simulink model "TST_Tra_Add"  (R2016b)
settings: Solver=FixedStepDiscrete  StartTime=0.0  StopTime=simTime  FixedStep=sampleTime  RelTol=1e-3
values from neighbouring files (symbols this model uses):
  testCase = 1    [initTST_Tra_Add_001.m]    (also in initTST_Tra_Add_002.m = 2)
libraries: simulink x7, UnitTest_Lib x4
settings Model: Creator=zhengjinyan  LastModifiedBy=zhengjinyan
settings DebuggingCC: SignalRangeChecking=error

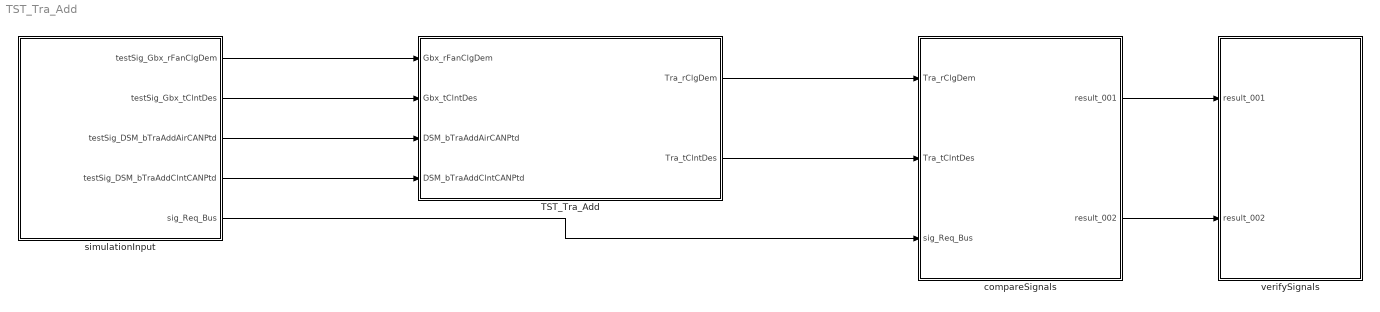
== system TST_Tra_Add ==
  TST_Tra_Add : Subsystem
  compareSignals : Subsystem
  simulationInput : Subsystem
  verifySignals : Subsystem
  wires:
  simulationInput/1(testSig_Gbx_rFanClgDem) -> TST_Tra_Add/1(Gbx_rFanClgDem)
  simulationInput/2(testSig_Gbx_tClntDes) -> TST_Tra_Add/2(Gbx_tClntDes)
  simulationInput/3(testSig_DSM_bTraAddAirCANPtd) -> TST_Tra_Add/3(DSM_bTraAddAirCANPtd)
  simulationInput/4(testSig_DSM_bTraAddClntCANPtd) -> TST_Tra_Add/4(DSM_bTraAddClntCANPtd)
  TST_Tra_Add/1(Tra_rClgDem) -> compareSignals/1(Tra_rClgDem)
  TST_Tra_Add/2(Tra_tClntDes) -> compareSignals/2(Tra_tClntDes)
  simulationInput/5(sig_Req_Bus) -> compareSignals/3(sig_Req_Bus)
  compareSignals/1(result_001) -> verifySignals/1(result_001)
  compareSignals/2(result_002) -> verifySignals/2(result_002)

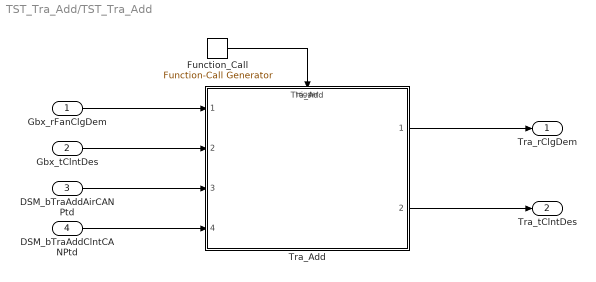
== system TST_Tra_Add/TST_Tra_Add ==
  Gbx_rFanClgDem : Inport
  Gbx_tClntDes : Inport  Port=2
  DSM_bTraAddAirCANPtd : Inport  Port=3
  DSM_bTraAddClntCANPtd : Inport  Port=4
  Function_Call : simulink/Ports & Subsystems/Function-Call Generator  sample_time=sampleTime  numberOfIterations=1
  Tra_Add : ModelReference  ModelNameDialog=Tra_Add  SimulationMode=Normal  ModelReferenceVersion=1.13  TriggerPortName=function  TriggerPortTriggerType=function-call  TriggerPortStatesWhenEnabling=held
  Tra_rClgDem : Outport
  Tra_tClntDes : Outport  Port=2
  wires:
  Function_Call/1 -> Tra_Add/Trigger
  Gbx_rFanClgDem/1 -> Tra_Add/1
  Gbx_tClntDes/1 -> Tra_Add/2
  DSM_bTraAddAirCANPtd/1 -> Tra_Add/3
  DSM_bTraAddClntCANPtd/1 -> Tra_Add/4
  Tra_Add/1 -> Tra_rClgDem/1
  Tra_Add/2 -> Tra_tClntDes/1

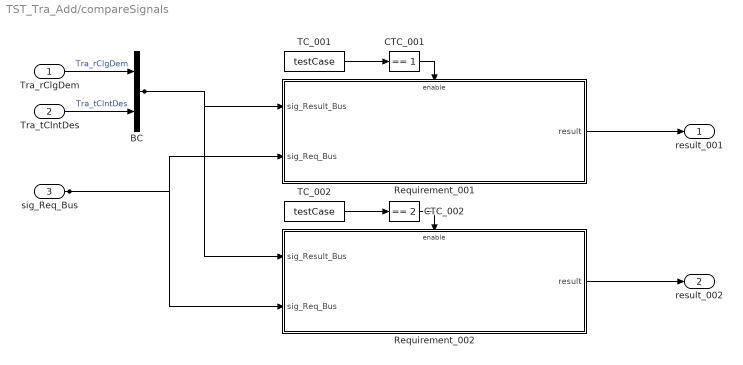
== system TST_Tra_Add/compareSignals ==
  Tra_rClgDem : Inport
  Tra_tClntDes : Inport  Port=2
  sig_Req_Bus : Inport  Port=3
  BC : BusCreator  Inputs=2
  CTC_001 : simulink/Logic and Bit Operations/Compare To Constant  relop===  const=1  OutDataTypeStr=boolean
  CTC_002 : simulink/Logic and Bit Operations/Compare To Constant  relop===  const=2  OutDataTypeStr=boolean
  Requirement_001 : Subsystem
  Requirement_002 : Subsystem
  TC_001 : Constant  Value=testCase
  TC_002 : Constant  Value=testCase
  result_001 : Outport
  result_002 : Outport  Port=2
  wires:
  Tra_rClgDem/1 -> BC/1  "Tra_rClgDem"
  Tra_tClntDes/1 -> BC/2  "Tra_tClntDes"
  TC_001/1 -> CTC_001/1
  CTC_001/1 -> Requirement_001/Enable
  sig_Req_Bus/1 -> Requirement_001/2(sig_Req_Bus), Requirement_002/2(sig_Req_Bus)
  BC/1 -> Requirement_001/1(sig_Result_Bus), Requirement_002/1(sig_Result_Bus)
  Requirement_001/1(result) -> result_001/1
  TC_002/1 -> CTC_002/1
  CTC_002/1 -> Requirement_002/Enable
  Requirement_002/1(result) -> result_002/1

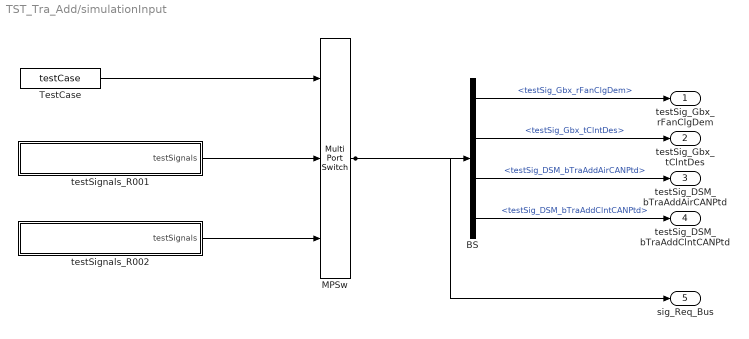
== system TST_Tra_Add/simulationInput ==
  BS : BusSelector  OutputSignals=testSig_Gbx_rFanClgDem,testSig_Gbx_tClntDes,testSig_DSM_bTraAddAirCANPtd,testSig_DSM_bTraAddClntCANPtd
  MPSw : MultiPortSwitch  Inputs=2  SaturateOnIntegerOverflow=on  InputSameDT=on
  TestCase : Constant  Value=testCase
  testSignals_R001 : Subsystem
  testSignals_R002 : Subsystem
  testSig_Gbx_rFanClgDem : Outport
  testSig_Gbx_tClntDes : Outport  Port=2
  testSig_DSM_bTraAddAirCANPtd : Outport  Port=3
  testSig_DSM_bTraAddClntCANPtd : Outport  Port=4
  sig_Req_Bus : Outport  Port=5
  wires:
  BS/1 -> testSig_Gbx_rFanClgDem/1  "<testSig_Gbx_rFanClgDem>"
  BS/2 -> testSig_Gbx_tClntDes/1  "<testSig_Gbx_tClntDes>"
  BS/3 -> testSig_DSM_bTraAddAirCANPtd/1  "<testSig_DSM_bTraAddAirCANPtd>"
  BS/4 -> testSig_DSM_bTraAddClntCANPtd/1  "<testSig_DSM_bTraAddClntCANPtd>"
  MPSw/1 -> BS/1, sig_Req_Bus/1
  TestCase/1 -> MPSw/1
  testSignals_R001/1(testSignals) -> MPSw/2
  testSignals_R002/1(testSignals) -> MPSw/3

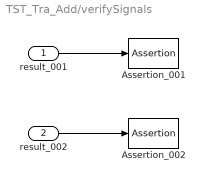
== system TST_Tra_Add/verifySignals ==
  result_001 : Inport
  result_002 : Inport  Port=2
  Assertion_001 : Assertion  Enabled=off
  Assertion_002 : Assertion  Enabled=off
  wires:
  result_001/1 -> Assertion_001/1
  result_002/1 -> Assertion_002/1

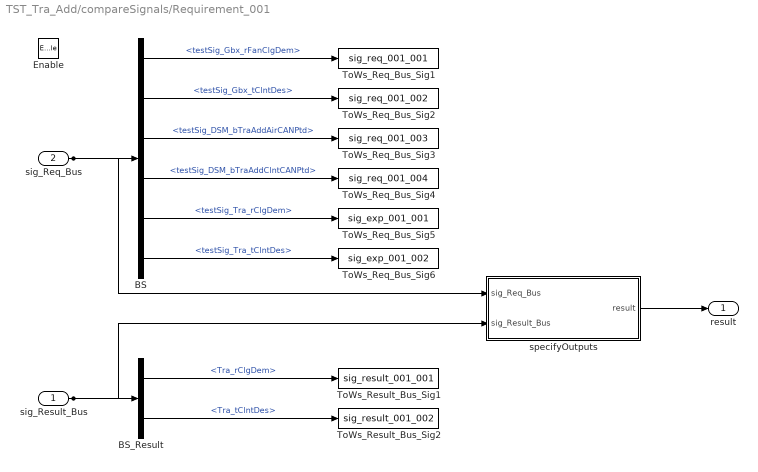
== system TST_Tra_Add/compareSignals/Requirement_001 ==
  sig_Result_Bus : Inport
  sig_Req_Bus : Inport  Port=2
  Enable : EnablePort
  BS : BusSelector  OutputSignals=testSig_Gbx_rFanClgDem,testSig_Gbx_tClntDes,testSig_DSM_bTraAddAirCANPtd,testSig_DSM_bTraAddClntCANPtd,testSig_Tra_rClgDem,testSig_Tra_tClntDes
  BS_Result : BusSelector  OutputSignals=Tra_rClgDem,Tra_tClntDes
  ToWs_Req_Bus_Sig1 : ToWorkspace  VariableName=sig_req_001_001  SaveFormat=Structure With Time
  ToWs_Req_Bus_Sig2 : ToWorkspace  VariableName=sig_req_001_002  SaveFormat=Structure With Time
  ToWs_Req_Bus_Sig3 : ToWorkspace  VariableName=sig_req_001_003  SaveFormat=Structure With Time
  ToWs_Req_Bus_Sig4 : ToWorkspace  VariableName=sig_req_001_004  SaveFormat=Structure With Time
  ToWs_Req_Bus_Sig5 : ToWorkspace  VariableName=sig_exp_001_001  SaveFormat=Structure With Time
  ToWs_Req_Bus_Sig6 : ToWorkspace  VariableName=sig_exp_001_002  SaveFormat=Structure With Time
  ToWs_Result_Bus_Sig1 : ToWorkspace  VariableName=sig_result_001_001  SaveFormat=Structure With Time
  ToWs_Result_Bus_Sig2 : ToWorkspace  VariableName=sig_result_001_002  SaveFormat=Structure With Time
  specifyOutputs : Subsystem
  result : Outport
  wires:
  sig_Req_Bus/1 -> BS/1, specifyOutputs/1(sig_Req_Bus)
  BS/1 -> ToWs_Req_Bus_Sig1/1  "<testSig_Gbx_rFanClgDem>"
  BS/2 -> ToWs_Req_Bus_Sig2/1  "<testSig_Gbx_tClntDes>"
  BS/3 -> ToWs_Req_Bus_Sig3/1  "<testSig_DSM_bTraAddAirCANPtd>"
  BS/4 -> ToWs_Req_Bus_Sig4/1  "<testSig_DSM_bTraAddClntCANPtd>"
  BS/5 -> ToWs_Req_Bus_Sig5/1  "<testSig_Tra_rClgDem>"
  BS/6 -> ToWs_Req_Bus_Sig6/1  "<testSig_Tra_tClntDes>"
  sig_Result_Bus/1 -> BS_Result/1, specifyOutputs/2(sig_Result_Bus)
  BS_Result/1 -> ToWs_Result_Bus_Sig1/1  "<Tra_rClgDem>"
  BS_Result/2 -> ToWs_Result_Bus_Sig2/1  "<Tra_tClntDes>"
  specifyOutputs/1(result) -> result/1

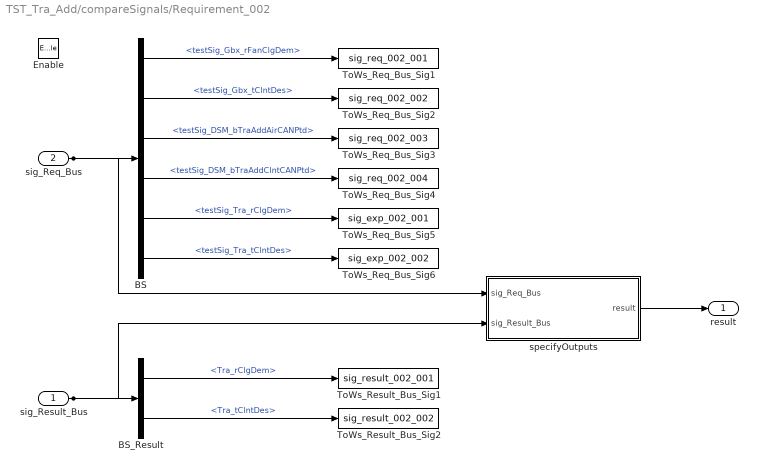
== system TST_Tra_Add/compareSignals/Requirement_002 ==
  sig_Result_Bus : Inport
  sig_Req_Bus : Inport  Port=2
  Enable : EnablePort
  BS : BusSelector  OutputSignals=testSig_Gbx_rFanClgDem,testSig_Gbx_tClntDes,testSig_DSM_bTraAddAirCANPtd,testSig_DSM_bTraAddClntCANPtd,testSig_Tra_rClgDem,testSig_Tra_tClntDes
  BS_Result : BusSelector  OutputSignals=Tra_rClgDem,Tra_tClntDes
  ToWs_Req_Bus_Sig1 : ToWorkspace  VariableName=sig_req_002_001  SaveFormat=Structure With Time
  ToWs_Req_Bus_Sig2 : ToWorkspace  VariableName=sig_req_002_002  SaveFormat=Structure With Time
  ToWs_Req_Bus_Sig3 : ToWorkspace  VariableName=sig_req_002_003  SaveFormat=Structure With Time
  ToWs_Req_Bus_Sig4 : ToWorkspace  VariableName=sig_req_002_004  SaveFormat=Structure With Time
  ToWs_Req_Bus_Sig5 : ToWorkspace  VariableName=sig_exp_002_001  SaveFormat=Structure With Time
  ToWs_Req_Bus_Sig6 : ToWorkspace  VariableName=sig_exp_002_002  SaveFormat=Structure With Time
  ToWs_Result_Bus_Sig1 : ToWorkspace  VariableName=sig_result_002_001  SaveFormat=Structure With Time
  ToWs_Result_Bus_Sig2 : ToWorkspace  VariableName=sig_result_002_002  SaveFormat=Structure With Time
  specifyOutputs : Subsystem
  result : Outport
  wires:
  sig_Req_Bus/1 -> BS/1, specifyOutputs/1(sig_Req_Bus)
  BS/1 -> ToWs_Req_Bus_Sig1/1  "<testSig_Gbx_rFanClgDem>"
  BS/2 -> ToWs_Req_Bus_Sig2/1  "<testSig_Gbx_tClntDes>"
  BS/3 -> ToWs_Req_Bus_Sig3/1  "<testSig_DSM_bTraAddAirCANPtd>"
  BS/4 -> ToWs_Req_Bus_Sig4/1  "<testSig_DSM_bTraAddClntCANPtd>"
  BS/5 -> ToWs_Req_Bus_Sig5/1  "<testSig_Tra_rClgDem>"
  BS/6 -> ToWs_Req_Bus_Sig6/1  "<testSig_Tra_tClntDes>"
  sig_Result_Bus/1 -> BS_Result/1, specifyOutputs/2(sig_Result_Bus)
  BS_Result/1 -> ToWs_Result_Bus_Sig1/1  "<Tra_rClgDem>"
  BS_Result/2 -> ToWs_Result_Bus_Sig2/1  "<Tra_tClntDes>"
  specifyOutputs/1(result) -> result/1

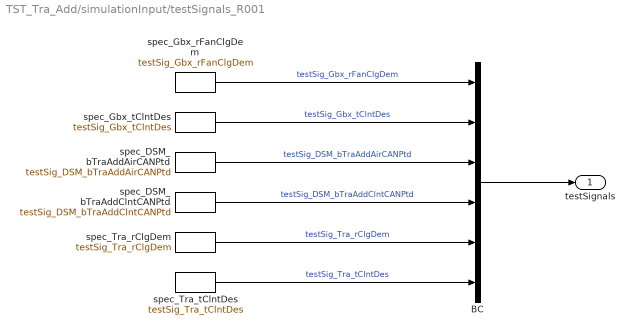
== system TST_Tra_Add/simulationInput/testSignals_R001 ==
  BC : BusCreator  Inputs=6
  spec_DSM_bTraAddAirCANPtd : FromWorkspace  VariableName=testSig_DSM_bTraAddAirCANPtd  Interpolate=off  OutputAfterFinalValue=Holding final value
  spec_DSM_bTraAddClntCANPtd : FromWorkspace  VariableName=testSig_DSM_bTraAddClntCANPtd  Interpolate=off  OutputAfterFinalValue=Holding final value
  spec_Gbx_rFanClgDem : FromWorkspace  VariableName=testSig_Gbx_rFanClgDem  Interpolate=off  OutputAfterFinalValue=Holding final value
  spec_Gbx_tClntDes : FromWorkspace  VariableName=testSig_Gbx_tClntDes  Interpolate=off  OutputAfterFinalValue=Holding final value
  spec_Tra_rClgDem : FromWorkspace  VariableName=testSig_Tra_rClgDem  Interpolate=off  OutputAfterFinalValue=Holding final value
  spec_Tra_tClntDes : FromWorkspace  VariableName=testSig_Tra_tClntDes  Interpolate=off  OutputAfterFinalValue=Holding final value
  testSignals : Outport
  wires:
  BC/1 -> testSignals/1
  spec_Gbx_rFanClgDem/1 -> BC/1  "testSig_Gbx_rFanClgDem"
  spec_Gbx_tClntDes/1 -> BC/2  "testSig_Gbx_tClntDes"
  spec_DSM_bTraAddAirCANPtd/1 -> BC/3  "testSig_DSM_bTraAddAirCANPtd"
  spec_DSM_bTraAddClntCANPtd/1 -> BC/4  "testSig_DSM_bTraAddClntCANPtd"
  spec_Tra_rClgDem/1 -> BC/5  "testSig_Tra_rClgDem"
  spec_Tra_tClntDes/1 -> BC/6  "testSig_Tra_tClntDes"

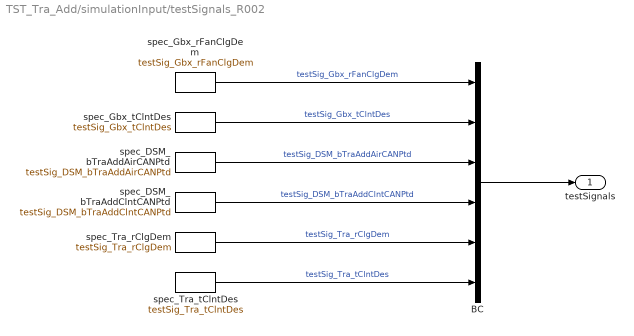
== system TST_Tra_Add/simulationInput/testSignals_R002 ==
  BC : BusCreator  Inputs=6
  spec_DSM_bTraAddAirCANPtd : FromWorkspace  VariableName=testSig_DSM_bTraAddAirCANPtd  Interpolate=off  OutputAfterFinalValue=Holding final value
  spec_DSM_bTraAddClntCANPtd : FromWorkspace  VariableName=testSig_DSM_bTraAddClntCANPtd  Interpolate=off  OutputAfterFinalValue=Holding final value
  spec_Gbx_rFanClgDem : FromWorkspace  VariableName=testSig_Gbx_rFanClgDem  Interpolate=off  OutputAfterFinalValue=Holding final value
  spec_Gbx_tClntDes : FromWorkspace  VariableName=testSig_Gbx_tClntDes  Interpolate=off  OutputAfterFinalValue=Holding final value
  spec_Tra_rClgDem : FromWorkspace  VariableName=testSig_Tra_rClgDem  Interpolate=off  OutputAfterFinalValue=Holding final value
  spec_Tra_tClntDes : FromWorkspace  VariableName=testSig_Tra_tClntDes  Interpolate=off  OutputAfterFinalValue=Holding final value
  testSignals : Outport
  wires:
  BC/1 -> testSignals/1
  spec_Gbx_rFanClgDem/1 -> BC/1  "testSig_Gbx_rFanClgDem"
  spec_Gbx_tClntDes/1 -> BC/2  "testSig_Gbx_tClntDes"
  spec_DSM_bTraAddAirCANPtd/1 -> BC/3  "testSig_DSM_bTraAddAirCANPtd"
  spec_DSM_bTraAddClntCANPtd/1 -> BC/4  "testSig_DSM_bTraAddClntCANPtd"
  spec_Tra_rClgDem/1 -> BC/5  "testSig_Tra_rClgDem"
  spec_Tra_tClntDes/1 -> BC/6  "testSig_Tra_tClntDes"

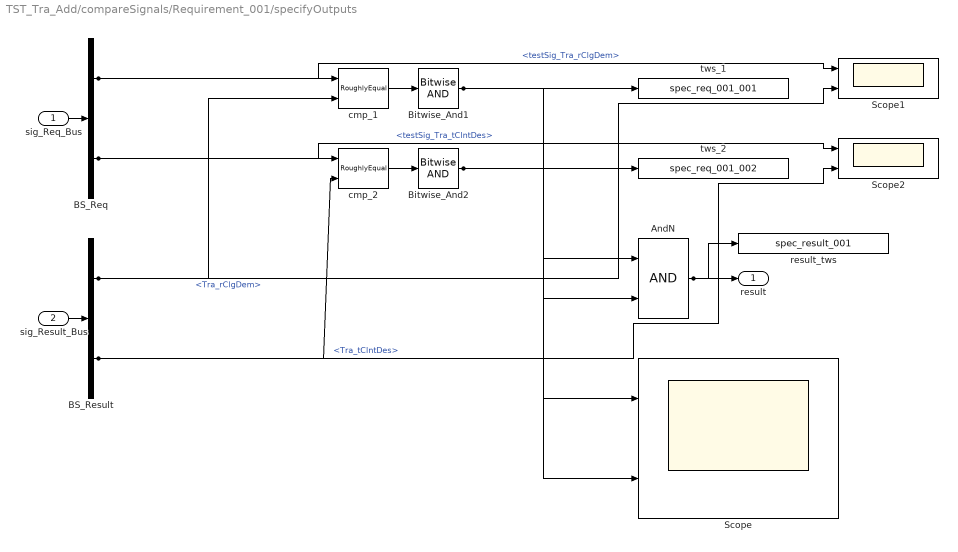
== system TST_Tra_Add/compareSignals/Requirement_001/specifyOutputs ==
  sig_Req_Bus : Inport
  sig_Result_Bus : Inport  Port=2
  AndN : Logic
  BS_Req : BusSelector  OutputSignals=testSig_Tra_rClgDem,testSig_Tra_tClntDes
  BS_Result : BusSelector  OutputSignals=Tra_rClgDem,Tra_tClntDes
  Bitwise_And1 : simulink/Logic and Bit Operations/Bitwise Operator  logicop=AND  UseBitMask=off  BitMask=bin2dec('11011001')  BitMaskRealWorld=Stored Integer
  Bitwise_And2 : simulink/Logic and Bit Operations/Bitwise Operator  logicop=AND  UseBitMask=off  BitMask=bin2dec('11011001')  BitMaskRealWorld=Stored Integer
  Scope : Scope  NumInputPorts=2
  Scope1 : Scope  NumInputPorts=2
  Scope2 : Scope  NumInputPorts=2
  cmp_1 : UnitTest_Lib/RoughlyEqual  slope=0.1
  cmp_2 : UnitTest_Lib/RoughlyEqual  slope=0.1
  result_tws : ToWorkspace  VariableName=spec_result_001
  tws_1 : ToWorkspace  VariableName=spec_req_001_001
  tws_2 : ToWorkspace  VariableName=spec_req_001_002
  result : Outport
  wires:
  sig_Req_Bus/1 -> BS_Req/1
  sig_Result_Bus/1 -> BS_Result/1
  AndN/1 -> result/1, result_tws/1
  BS_Req/1 -> cmp_1/1, Scope1/1  "<testSig_Tra_rClgDem>"
  BS_Result/1 -> cmp_1/2, Scope1/2  "<Tra_rClgDem>"
  cmp_1/1 -> Bitwise_And1/1
  Bitwise_And1/1 -> tws_1/1, AndN/1, Scope/1
  BS_Req/2 -> cmp_2/1, Scope2/1  "<testSig_Tra_tClntDes>"
  BS_Result/2 -> cmp_2/2, Scope2/2  "<Tra_tClntDes>"
  cmp_2/1 -> Bitwise_And2/1
  Bitwise_And2/1 -> tws_2/1, AndN/2, Scope/2

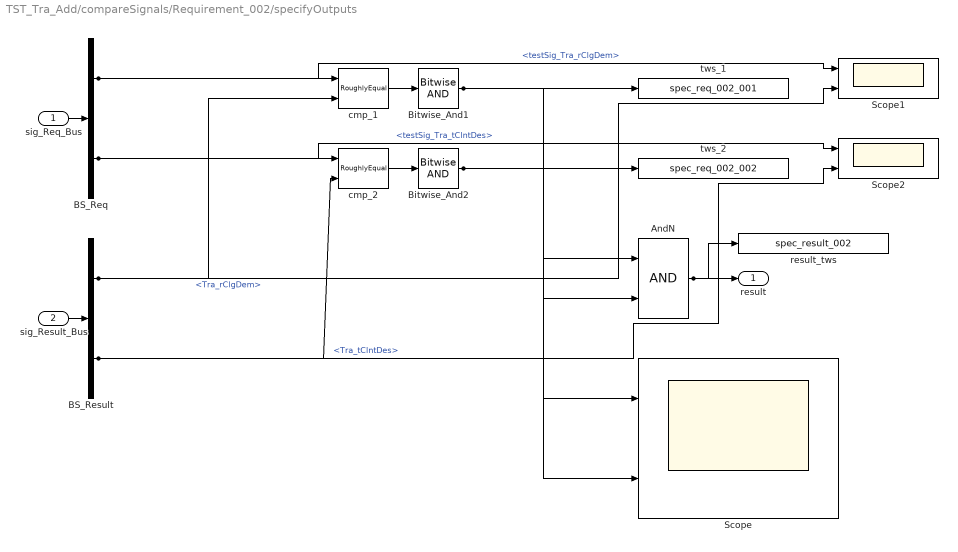
== system TST_Tra_Add/compareSignals/Requirement_002/specifyOutputs ==
  sig_Req_Bus : Inport
  sig_Result_Bus : Inport  Port=2
  AndN : Logic
  BS_Req : BusSelector  OutputSignals=testSig_Tra_rClgDem,testSig_Tra_tClntDes
  BS_Result : BusSelector  OutputSignals=Tra_rClgDem,Tra_tClntDes
  Bitwise_And1 : simulink/Logic and Bit Operations/Bitwise Operator  logicop=AND  UseBitMask=off  BitMask=bin2dec('11011001')  BitMaskRealWorld=Stored Integer
  Bitwise_And2 : simulink/Logic and Bit Operations/Bitwise Operator  logicop=AND  UseBitMask=off  BitMask=bin2dec('11011001')  BitMaskRealWorld=Stored Integer
  Scope : Scope  NumInputPorts=2
  Scope1 : Scope  NumInputPorts=2
  Scope2 : Scope  NumInputPorts=2
  cmp_1 : UnitTest_Lib/RoughlyEqual  slope=0.1
  cmp_2 : UnitTest_Lib/RoughlyEqual  slope=0.1
  result_tws : ToWorkspace  VariableName=spec_result_002
  tws_1 : ToWorkspace  VariableName=spec_req_002_001
  tws_2 : ToWorkspace  VariableName=spec_req_002_002
  result : Outport
  wires:
  sig_Req_Bus/1 -> BS_Req/1
  sig_Result_Bus/1 -> BS_Result/1
  AndN/1 -> result/1, result_tws/1
  BS_Req/1 -> cmp_1/1, Scope1/1  "<testSig_Tra_rClgDem>"
  BS_Result/1 -> cmp_1/2, Scope1/2  "<Tra_rClgDem>"
  cmp_1/1 -> Bitwise_And1/1
  Bitwise_And1/1 -> tws_1/1, AndN/1, Scope/1
  BS_Req/2 -> cmp_2/1, Scope2/1  "<testSig_Tra_tClntDes>"
  BS_Result/2 -> cmp_2/2, Scope2/2  "<Tra_tClntDes>"
  cmp_2/1 -> Bitwise_And2/1
  Bitwise_And2/1 -> tws_2/1, AndN/2, Scope/2
